simulink model "test"  (R2019a)
settings: Solver=VariableStepAuto  StartTime=0.0  StopTime=10.0  RelTol=1e-3
values from neighbouring files (symbols this model uses):
  a = [0.328350063485 -0.504393436497 -18.7824329195 1.02511531984 -53.4041424252]    [a.mat]    (also in a1.mat = [-0.685212439995 -0.585400025674 -24.4194734415 0.9475851353; a2.mat = [-1.28043820376 -0.621828624231 -54.7528450797 1.71837449641; system_id.m = pinv(G1'*G1)*G1'*E)
  b = [6.12465019513 -5.20663579301 6.03715613869 77.417940964 10.1407211952]    [b.mat]    (also in b1.mat = [34.2019090673 -33.7070179637 52.7248095782 336.319136551 44; b2.mat = [16.939936533 -14.6014953721 67.1462611587 436.465012222 564; system_id.m = pinv(G2'*G2)*G2'*E)
undefined symbols (not defined in the file or in its folder): DiscIntNeverNeededParam
settings Model: Creator=ray  LastModifiedBy=ASUS
settings DebuggingCC: AlgebraicLoopMsg=none

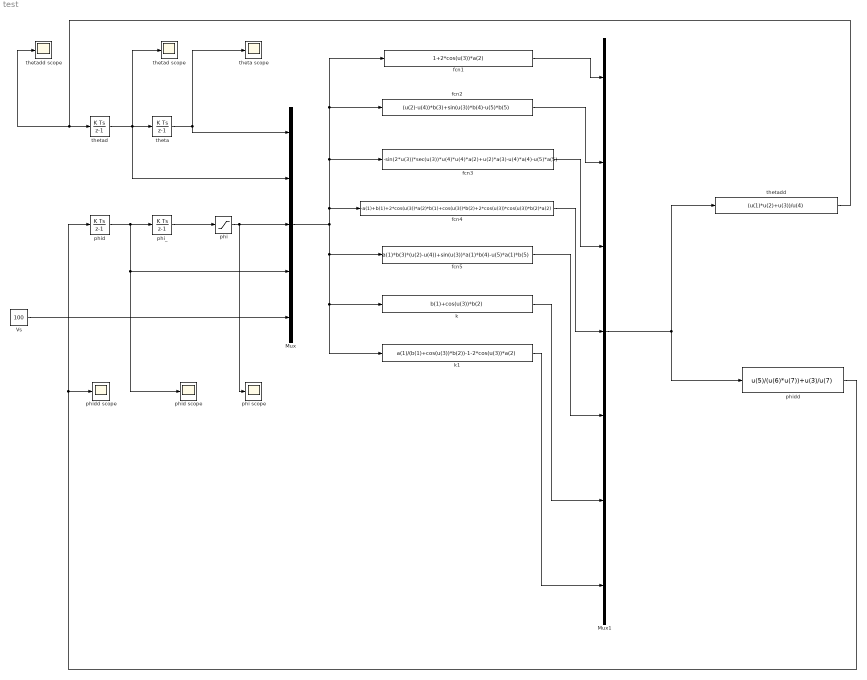
== system test ==
  Mux : Mux  Inputs=5
  Mux1 : Mux  Inputs=7
  Vs : Constant  Value=100
  fcn1 : Fcn  Expr=1+2*cos(u(3))*a(2)
  fcn2 : Fcn  Expr=(u(2)-u(4))*b(3)+sin(u(3))*b(4)-u(5)*b(5)
  fcn3 : Fcn  Expr=-sin(2*u(3))*sec(u(3))*u(4)*u(4)*a(2)+u(2)*a(3)-u(4)*a(4)-u(5)*a(5)
  fcn4 : Fcn  Expr=-a(1)+b(1)+2*cos(u(3))*a(2)*b(1)+cos(u(3))*b(2)+2*cos(u(3))*cos(u(3))*b(2)*a(2)
  fcn5 : Fcn  Expr=a(1)*b(3)*(u(2)-u(4))+sin(u(3))*a(1)*b(4)-u(5)*a(1)*b(5)
  k : Fcn  Expr=b(1)+cos(u(3))*b(2)
  k1 : Fcn  Expr=a(1)/(b(1)+cos(u(3))*b(2))-1-2*cos(u(3))*a(2)
  phi : Saturate  UpperLimit=1.6  LowerLimit=-1.6
  "phi scope " : Scope
  phi_ : DiscreteIntegrator  InitialCondition=pi/180  SampleTime=0.001  ICPrevOutput=DiscIntNeverNeededParam  ICPrevScaledInput=DiscIntNeverNeededParam
  phid : DiscreteIntegrator  InitialCondition=0.1  SampleTime=0.001  ICPrevOutput=DiscIntNeverNeededParam  ICPrevScaledInput=DiscIntNeverNeededParam
  "phid scope " : Scope
  phidd : Fcn  Expr=u(5)/(u(6)*u(7))+u(3)/u(7)
  "phidd scope " : Scope
  theta : DiscreteIntegrator  SampleTime=0.001  ICPrevOutput=DiscIntNeverNeededParam  ICPrevScaledInput=DiscIntNeverNeededParam
  theta scope : Scope
  thetad : DiscreteIntegrator  SampleTime=0.001  ICPrevOutput=DiscIntNeverNeededParam  ICPrevScaledInput=DiscIntNeverNeededParam
  "thetad scope " : Scope
  thetadd : Fcn  Expr=(u(1)*u(2)+u(3))/u(4)
  "thetadd scope " : Scope
  wires:
  phid/1 -> Mux/4, "phid scope "/1, phi_/1
  phi_/1 -> phi/1
  phi/1 -> Mux/3, "phi scope "/1
  phidd/1 -> "phidd scope "/1, phid/1
  Vs/1 -> Mux/5
  fcn5/1 -> Mux1/5
  fcn4/1 -> Mux1/4
  fcn3/1 -> Mux1/3
  fcn2/1 -> Mux1/2
  fcn1/1 -> Mux1/1
  theta/1 -> theta scope/1, Mux/1
  Mux1/1 -> thetadd/1, phidd/1
  Mux/1 -> fcn1/1, fcn2/1, fcn3/1, fcn4/1, k1/1, k/1, fcn5/1
  thetad/1 -> "thetad scope "/1, Mux/2, theta/1
  thetadd/1 -> "thetadd scope "/1, thetad/1
  k/1 -> Mux1/6
  k1/1 -> Mux1/7
